simulink model "ccode_sdr"  (Simulink 8.1)
settings: Solver=ode45  StartTime=0.0  StopTime=10000  RelTol=1e-3
libraries: simulink x2, commchan3 x1, commdigbbndpm3 x1, commrandsrc2 x1
settings Model: Creator=Gaurav  LastModifiedBy=Gaurav
settings DataIOCC: SignalLoggingSaveFormat=Dataset
settings OptimizationCC: ExpressionDepthLimit=128
settings DebuggingCC: FcnCallInpInsideContextMsg=EnableAllAsError
settings GRTTargetCC: CombineOutputUpdateFcns=on  GRTInterface=off

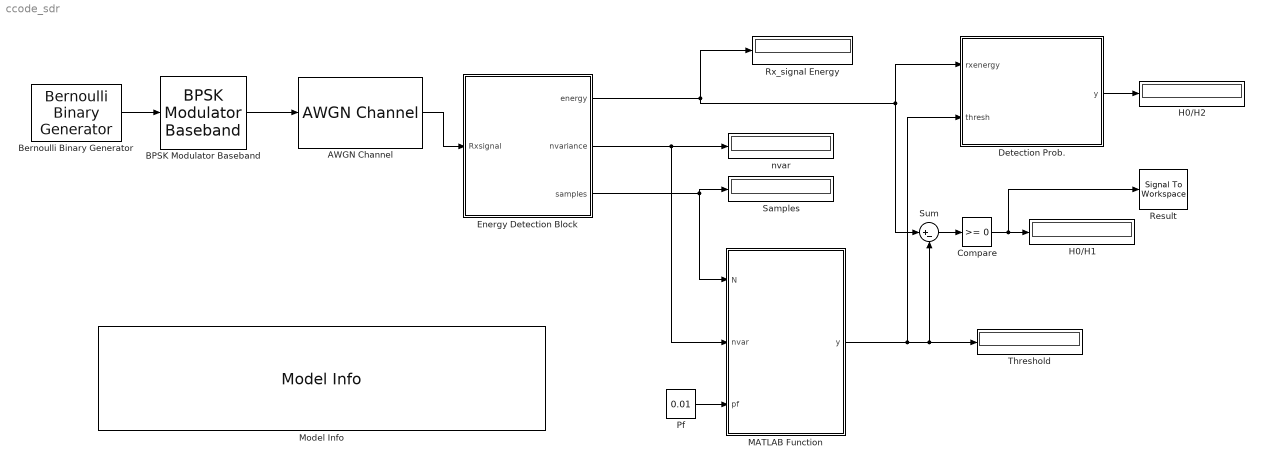
== system ccode_sdr ==
  AWGN Channel : commchan3/AWGN Channel  InputProcessing=Columns as channels (frame based)  seed=67  noiseMode="Signal to noise ratio  (SNR)"  EbNodB=10  EsNodB=10  SNRdB=-10  bitsPerSym=1  Ps=1  Tsym=1  variance=1
  BPSK Modulator Baseband : commdigbbndpm3/BPSK Modulator Baseband  Ph=0  outDtype=double  outWordLen=16  outUDDataType=sfix(16)  outFracLenMode=Best precision  outFracLen=15
  Bernoulli Binary Generator : commrandsrc2/Bernoulli Binary Generator  P=0.5  seed=90  Ts=0.01  frameBased=on  sampPerFrame=1000  orient=off  outDataType=double
  Compare : simulink/Logic and Bit Operations/Compare To Zero  relop=>=  OutDataTypeStr=boolean
  Detection Prob. : MATLAB Function  TreatAsAtomicUnit=on
  "Energy Detection Block " : Subsystem
  H0/H1 : Display
  H0/H2 : Display
  MATLAB Function : MATLAB Function  TreatAsAtomicUnit=on
  Model Info : simulink/Model-Wide Utilities/Model Info  InitialBlockCM=None  BlockCM=None  Frame=on  DisplayStringWithTags=|  HorizontalTextAlignment=Center  LeftAlignmentValue=0.5  SourceBlockDiagram=ccode_sdr  TagMaxNumber=20
      | Gaurav Sharma
      | %<ModifiedDate>
      | Energy Detection
      | Model Run from RunSDR .m file
      | %<LastModificationDate>
  Pf : Constant  Value=0.01
  Result : SignalToWorkspace  VariableName=Stat
      settings: CopyFcn=dspblkcopystw(gcbh);
  Rx_signal Energy : Display
  Samples : Display
  Sum : Sum  Inputs=|+-
  Threshold : Display
  nvar : Display
  wires:
  Bernoulli Binary Generator/1 -> BPSK Modulator Baseband/1
  BPSK Modulator Baseband/1 -> AWGN Channel/1
  Pf/1 -> MATLAB Function/3(pf)
  MATLAB Function/1(y) -> Detection Prob./2(thresh), Threshold/1, Sum/2
  Sum/1 -> Compare/1
  Compare/1 -> Result/1, H0/H1/1
  Detection Prob./1(y) -> H0/H2/1
  "Energy Detection Block "/3(samples) -> MATLAB Function/1(N), Samples/1
  "Energy Detection Block "/2(nvariance) -> MATLAB Function/2(nvar), nvar/1
  "Energy Detection Block "/1(energy) -> Sum/1, Detection Prob./1(rxenergy), Rx_signal Energy/1
  AWGN Channel/1 -> "Energy Detection Block "/1(Rxsignal)

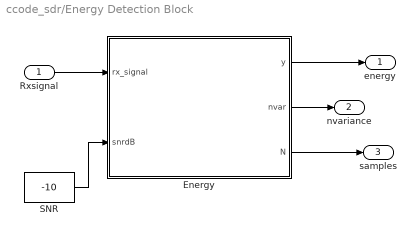
== system ccode_sdr/Energy Detection Block  ==
  Rxsignal : Inport
  Energy : MATLAB Function  TreatAsAtomicUnit=on
  SNR : Constant  Value=-10
  energy : Outport
  nvariance : Outport  Port=2
  samples : Outport  Port=3
  wires:
  Rxsignal/1 -> Energy/1(rx_signal)
  SNR/1 -> Energy/2(snrdB)
  Energy/1(y) -> energy/1
  Energy/3(N) -> samples/1
  Energy/2(nvar) -> nvariance/1

== matlab function MATLAB Function ==
  data: N input double; y output double; nvar input double; pf input double
function y = Threshold(N,nvar,pf)
    coder.extrinsic('qfuncinv');
    t=double(zeros(1,1));
    t=qfuncinv(pf);
    thresh=double(zeros(1,1));
    thresh = sqrt(2*N*nvar^4)*t+N*nvar^2;
y=thresh;

== matlab function Energy Detection Block /Energy ==
  data: rx_signal input double; y output double; snrdB input double; nvar output double; N output double
function [y,nvar,N] = Energy(rx_signal,snrdB)
    [n,m]=size(rx_signal);
    %energy=double(zeros(1,1));
    energy = sum(abs(rx_signal).^2); 
    snr = 10^(snrdB/20);
    nvar = 1/snr;                               % noise variance
    y = energy;
    N=n;

== matlab function Detection Prob. ==
  data: rxenergy input double; y output double; thresh input double
function y = Detectionprob(rxenergy,thresh)
       t=double(zeros(1,1));
       if(rxenergy>=thresh)
           t=t+1;
       end
%     [p q]=size(R);
%     detect=double(zeros(1,1));
%     for i=1:p
%         p
%         if(R(p,1)==1)
%             detect=detect+1;
%             detect
%         end
%     end
y = t;
